simulink model "RetinaGuard_SimEvents_Day2"  (R2026a)
settings: Solver=VariableStepAuto  StopTime=480
InitFcn:
  | init_retinaguard_day2
undefined symbols (not defined in the file): m, n
settings Model: Creator=NITIN  LastModifiedBy=Dell

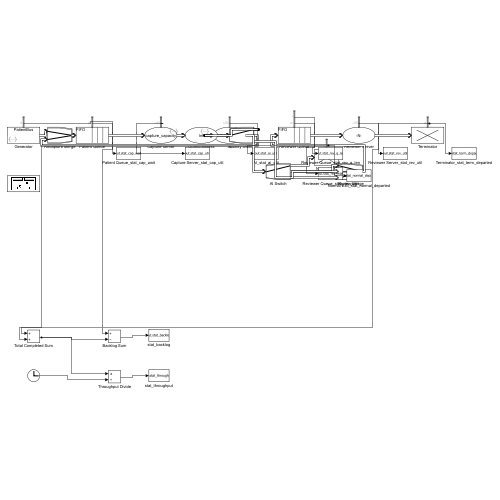
[thumbnail: Simulink's stored preview of the top-level diagram]
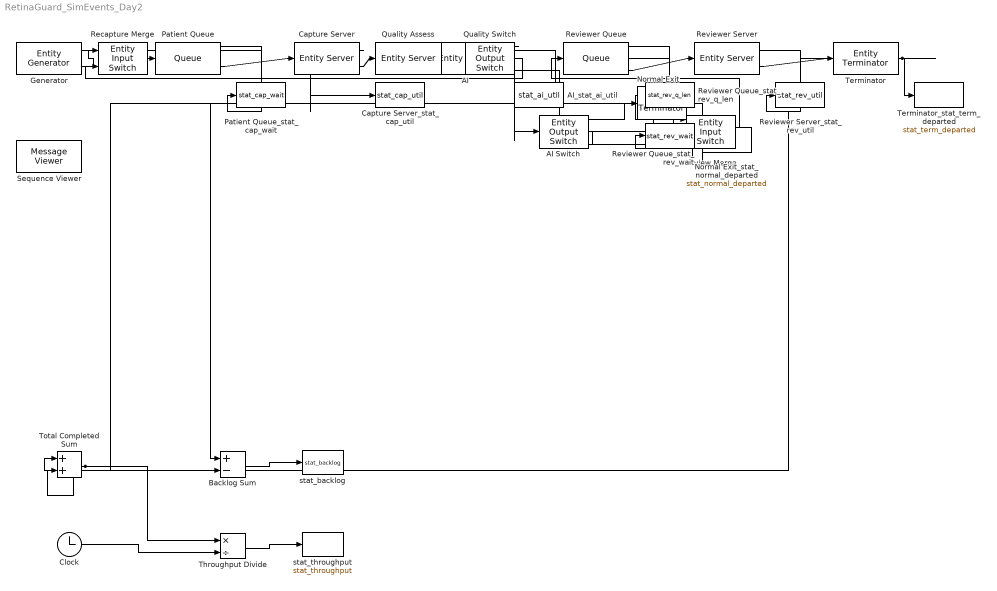
== system RetinaGuard_SimEvents_Day2 ==
  AI : EntityServer  InputPortMessageModes=m  OutputPortMessageModes=n,m  Capacity=1  ServiceTimeValue=ai_svc_t  EntryAction=|  Utilization=on
      | r = rand();
      | if r < p_normal
      |     entity.AIResult = 1;
      | elseif r < p_normal + p_referable
      |     entity.AIResult = 2;
      | else
      |     entity.AIResult = 3;
      | end
      settings: OutputPortMap=o5,o9
  AI Switch : EntityOutputSwitch  InputPortMessageModes=m  OutputPortMessageModes=m,m,m  NumberOutputPorts=3  SwitchingCriterion=From attribute  SwitchAttributeName=AIResult
      settings: OutputPortMap=o0,o1,o2
  AI_stat_ai_util : ToWorkspace  VariableName=stat_ai_util  SaveFormat=Timeseries  SampleTime=-1
  Backlog Sum : Sum  Inputs=+-
  Capture Server : EntityServer  InputPortMessageModes=m  OutputPortMessageModes=n,m  Capacity=capture_capacity  ServiceTimeValue=capture_svc_t  Utilization=on
      settings: OutputPortMap=o5,o9
  Capture Server_stat_cap_util : ToWorkspace  VariableName=stat_cap_util  SaveFormat=Timeseries  SampleTime=-1
  Clock : Clock
  Generator : EntityGenerator  OutputPortMessageModes=n,m  TimeSource=MATLAB action  IntergenerationTimeAction=|  GenerateAction=entity.AIResult = 0; entity.Attempts = 0; entity.Quality = 1;  NumberEntitiesDeparted=on  EntityType=Bus object  EntityTypeName=PatientBus
      | persistent init;
      | if isempty(init)
      |     seed = sim_seed;
      |     for i=1:seed; rand(); end
      |     init = true;
      | end
      | dt = -0.5 * log(rand());
      settings: OutputPortMap=o0,o3
  Normal Exit : EntityTerminator  InputPortMessageModes=m  NumberEntitiesArrived=on
      settings: OutputPortMap=o0
  Normal Exit_stat_normal_departed : ToWorkspace  VariableName=stat_normal_departed  SaveFormat=Timeseries  SampleTime=-1
  Patient Queue : Queue  InputPortMessageModes=m  OutputPortMessageModes=n,m  Capacity=500  AverageWait=on
      settings: OutputPortMap=o2,o5
  Patient Queue_stat_cap_wait : ToWorkspace  VariableName=stat_cap_wait  SaveFormat=Timeseries  SampleTime=-1
  Quality Assess : EntityServer  InputPortMessageModes=m  OutputPortMessageModes=m  Capacity=Inf  ServiceTimeValue=0  EntryAction=|
      | persistent init;
      | if isempty(init)
      |     seed = sim_seed + 1000;
      |     for i=1:seed; rand(); end
      |     init = true;
      | end
      | entity.Attempts = entity.Attempts + 1;
      | if entity.Attempts >= 2
      |     entity.Quality = 3;
      | elseif rand() < p_poor
      |     entity.Quality = 2;
      | else
      |     entity.Quality = 1;
      | end
  Quality Switch : EntityOutputSwitch  InputPortMessageModes=m  OutputPortMessageModes=m,m,m  NumberOutputPorts=3  SwitchingCriterion=From attribute  SwitchAttributeName=Quality
      settings: OutputPortMap=o0,o1,o2
  Recapture Merge : EntityInputSwitch  InputPortMessageModes=m,m  OutputPortMessageModes=m
  Review Merge : EntityInputSwitch  InputPortMessageModes=m,m,m  OutputPortMessageModes=m  NumberInputPorts=3
      settings: InputPortMap=u1,u2,u3
  Reviewer Queue : Queue  InputPortMessageModes=m  OutputPortMessageModes=n,n,m  Capacity=500  AverageWait=on  AverageQueueLength=on
      settings: OutputPortMap=o2,o3,o5
  Reviewer Queue_stat_rev_q_len : ToWorkspace  VariableName=stat_rev_q_len  SaveFormat=Timeseries  SampleTime=-1
  Reviewer Queue_stat_rev_wait : ToWorkspace  VariableName=stat_rev_wait  SaveFormat=Timeseries  SampleTime=-1
  Reviewer Server : EntityServer  InputPortMessageModes=m  OutputPortMessageModes=n,m  Capacity=reviewer_capacity  ServiceTimeValue=reviewer_svc_t  Utilization=on
      settings: OutputPortMap=o5,o9
  Reviewer Server_stat_rev_util : ToWorkspace  VariableName=stat_rev_util  SaveFormat=Timeseries  SampleTime=-1
  Sequence Viewer : MessageViewer  History=1000  SavedRootId=#
  Terminator : EntityTerminator  InputPortMessageModes=m  NumberEntitiesArrived=on
      settings: OutputPortMap=o0
  Terminator_stat_term_departed : ToWorkspace  VariableName=stat_term_departed  SaveFormat=Timeseries  SampleTime=-1
  Throughput Divide : Product  Inputs=*/
  Total Completed Sum : Sum
  stat_backlog : ToWorkspace  VariableName=stat_backlog  SaveFormat=Timeseries  SampleTime=-1
  stat_throughput : ToWorkspace  VariableName=stat_throughput  SaveFormat=Timeseries  SampleTime=-1
  wires:
  Patient Queue/2 -> Capture Server/1
  Reviewer Queue/3 -> Reviewer Server/1
  Reviewer Server/2 -> Terminator/1
  Generator/2 -> Recapture Merge/1
  Recapture Merge/1 -> Patient Queue/1
  Capture Server/2 -> Quality Assess/1
  Quality Assess/1 -> Quality Switch/1
  Quality Switch/1 -> AI/1
  Quality Switch/2 -> Recapture Merge/2
  Review Merge/1 -> Reviewer Queue/1
  Quality Switch/3 -> Review Merge/3
  AI/2 -> AI Switch/1
  AI Switch/1 -> Normal Exit/1
  AI Switch/2 -> Review Merge/1
  AI Switch/3 -> Review Merge/2
  Terminator/1 -> Terminator_stat_term_departed/1, Total Completed Sum/2
  Normal Exit/1 -> Normal Exit_stat_normal_departed/1, Total Completed Sum/1
  Capture Server/1 -> Capture Server_stat_cap_util/1
  AI/1 -> AI_stat_ai_util/1
  Reviewer Server/1 -> Reviewer Server_stat_rev_util/1
  Reviewer Queue/2 -> Reviewer Queue_stat_rev_q_len/1
  Reviewer Queue/1 -> Reviewer Queue_stat_rev_wait/1
  Patient Queue/1 -> Patient Queue_stat_cap_wait/1
  Total Completed Sum/1 -> Backlog Sum/2, Throughput Divide/1
  Backlog Sum/1 -> stat_backlog/1
  Clock/1 -> Throughput Divide/2
  Throughput Divide/1 -> stat_throughput/1
  Generator/1 -> Backlog Sum/1
